simulink model "METI_CVT_Thermal_ver01_2015a"  (R2015a)
settings: Solver=ode8  SolverMode=SingleTasking  StartTime=0  StopTime=1204  FixedStep=sampling_time  RelTol=1e-3
PreLoadFcn:
  | init_setting;
values from neighbouring files (symbols this model uses):
  degC2K = 273.15    [METI_TRAMI_Thermal_ver01_Jmaab_PreLoad.m]    (also in init_setting_METI.m)
  K2degC = -273.15    [METI_TRAMI_Thermal_ver01_Jmaab_PreLoad.m]    (also in init_setting_METI.m)
  sampling_time = 0.0025    [METI_TRAMI_Thermal_ver01_Jmaab_PreLoad.m]
undefined symbols (not defined in the file or in its folder): ALT_CNT_ALT_OFF_RPM_HYS_rpm, ALT_CNT_ALT_ON_RPM_HYS_rpm, ALT_CNT_Alter_V_BASE_V, ALT_CNT_Alter_V_Kaisei_V, ALT_CNT_flag_disable_kaisei, ALT_CNT_V_Battely_Kudo_V, ALT_PNT_ALT_GDCurrent_A, ALT_PNT_ALT_GDVolt_V, ALT_PNT_Alter_limit_Current_V_table, ALT_PNT_Alter_limit_Current_V_table_x_rpm, ALT_PNT_Alter_trq_Nm_map, ALT_PNT_Alter_trq_Nm_map_x_rpm, ALT_PNT_Alter_trq_Nm_map_y_Current_A, ALT_PNT_Alter_trq_Nm_map_z_Volt_tgt_V, ALT_PNT_eta_pulley_alt, ALT_PNT_Gain_Alt_v_del, ALT_PNT_ratio_pulley_alt, ALT_PNT_Tau_Alternator_V_tgt_s, ALT_PNT_trq_alter_output_LL_Nm, BK_PNT_Pow_UL, BK_PNT_Tau_brake, Brk_LL, Brk_PGain, Brk_UL, BT_PNT_Lo_Capa_lo_batt_F, BT_PNT_Lo_ocv_SOC_lo_batt_OCV_V_table, BT_PNT_Lo_ocv_SOC_lo_batt_OCV_V_table_x_SOC, BT_PNT_Lo_R_lo_batt_ohm, BT_PNT_Lo_SOC_MAX_lo_batt, BT_PNT_Lo_SOC_MIN_lo_batt, BT_PNT_Lo_SOC_START_lo_batt, DF_PNT_DF_gear, DF_PNT_DFBlock2DFAir_Heat_Resi_KpW, DF_PNT_DFBlock_Heat_Capa_JpK, DF_PNT_DFBlock_Temp_ini_degC, DF_PNT_DFOil2DFBlock_Heat_Resi_KpW, DF_PNT_DFOil_Heat_Capa_JpK, DF_PNT_DFOil_Temp_ini_degC, DF_PNT_Driveshaft_damper, DF_PNT_Driveshaft_delta_radps_LL, DF_PNT_Driveshaft_delta_radps_UL, DF_PNT_Driveshaft_spring, DF_PNT_eta_DF, DF_PNT_Outtemp_degC, DF_PNT_TMBlock2DFBlock_Heat_Resi_KpW, Driver_Brake_Const1, Driver_Brake_Const3, Driver_Brake_Switch_Const2, Driver_Brk_sh, drivmode_ACC, drivmode_CONST, drivmode_GensokuKaisei, drivmode_GensokuRikko, drivmode_STOP, EL_PNT_R_bodyelec_lo_ohm, ENG_CNT_acc_idlestop, ENG_CNT_Accel_LL, ENG_CNT_Accel_UL, ENG_CNT_brak_idlestop, ENG_CNT_flag_idle_stop_exe ... (+133)
undefined symbols (not defined in the file): ACC_D_Gain, ACC_I_Gain, ACC_P_Gain
libraries: METI_Lib_vehicle_model x32, simulink x7, AZAPA_Lib_vehicle_model x1
(part 2 of 3)

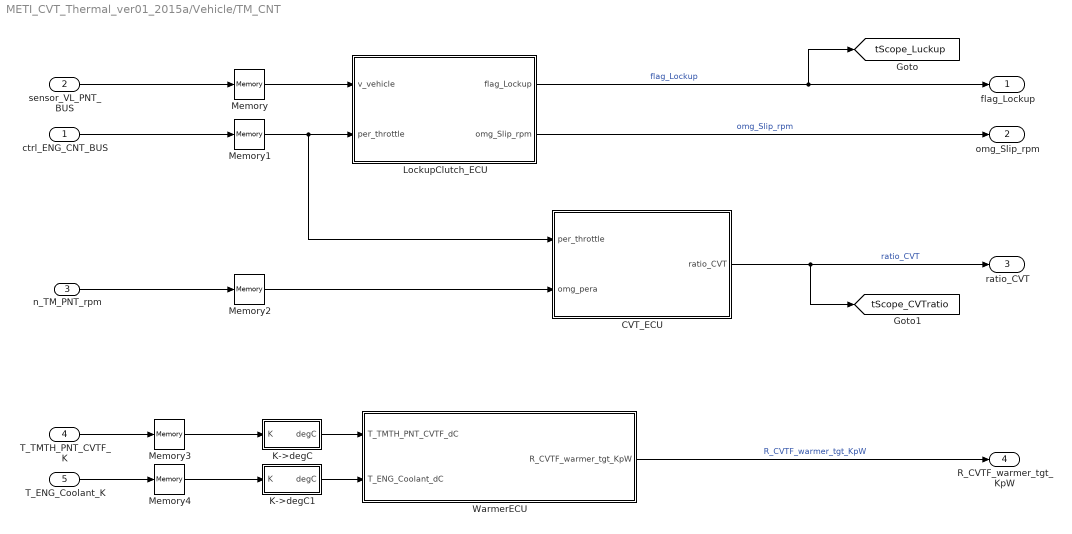
== system METI_CVT_Thermal_ver01_2015a/Vehicle/TM_CNT ==
  ctrl_ENG_CNT_BUS : Inport
  sensor_VL_PNT_BUS : Inport  Port=2
  n_TM_PNT_rpm : Inport  Port=3
  T_TMTH_PNT_CVTF_K : Inport  Port=4
  T_ENG_Coolant_K : Inport  Port=5
  CVT_ECU : Subsystem
  K->degC : Subsystem
  K->degC1 : Subsystem
  LockupClutch_ECU : Subsystem
  Memory{,1..4} (5 alike) : Memory
  WarmerECU : Subsystem
  flag_Lockup : Outport
  omg_Slip_rpm : Outport  Port=2
  ratio_CVT : Outport  Port=3
  R_CVTF_warmer_tgt_KpW : Outport  Port=4
  tag scope: tScope_CVTratio=global, tScope_Luckup=global
  wires:
  CVT_ECU/1(ratio_CVT) -> [tScope_CVTratio], ratio_CVT/1  "ratio_CVT"
  LockupClutch_ECU/1(flag_Lockup) -> [tScope_Luckup], flag_Lockup/1  "flag_Lockup"
  LockupClutch_ECU/2(omg_Slip_rpm) -> omg_Slip_rpm/1  "omg_Slip_rpm"
  ctrl_ENG_CNT_BUS/1 -> Memory1/1
  Memory/1 -> LockupClutch_ECU/1(v_vehicle)
  Memory1/1 -> CVT_ECU/1(per_throttle), LockupClutch_ECU/2(per_throttle)
  Memory2/1 -> CVT_ECU/2(omg_pera)
  n_TM_PNT_rpm/1 -> Memory2/1
  sensor_VL_PNT_BUS/1 -> Memory/1
  T_TMTH_PNT_CVTF_K/1 -> Memory3/1
  T_ENG_Coolant_K/1 -> Memory4/1
  Memory3/1 -> K->degC/1(K)
  Memory4/1 -> K->degC1/1(K)
  WarmerECU/1(R_CVTF_warmer_tgt_KpW) -> R_CVTF_warmer_tgt_KpW/1  "R_CVTF_warmer_tgt_KpW"
  K->degC/1(degC) -> WarmerECU/1(T_TMTH_PNT_CVTF_dC)
  K->degC1/1(degC) -> WarmerECU/2(T_ENG_Coolant_dC)

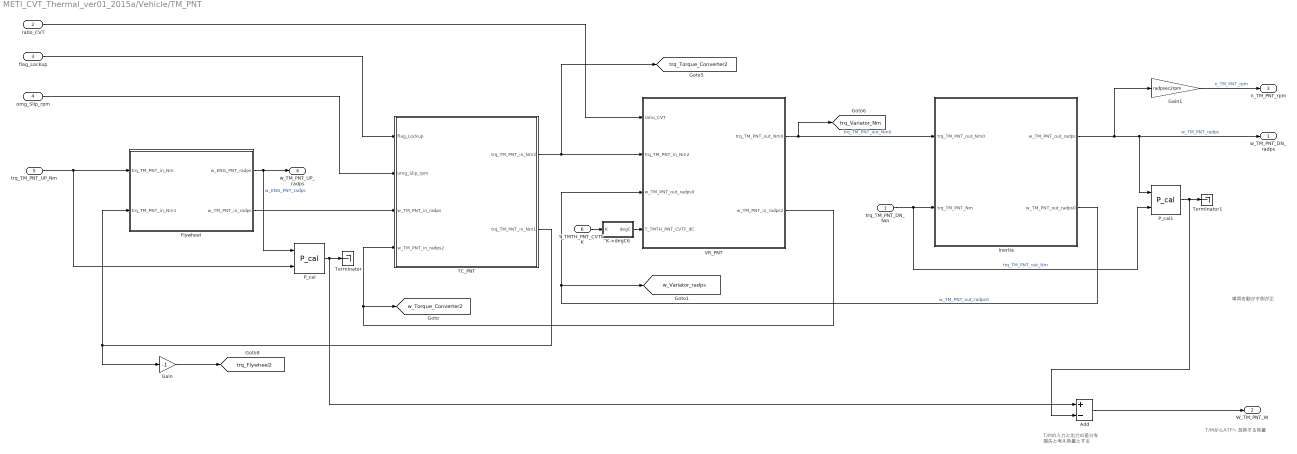
== system METI_CVT_Thermal_ver01_2015a/Vehicle/TM_PNT ==
  note: 車両を動かす側が正
  note: T/MからATFへ
      | 放熱する熱量
  note: T/Mの入力と出力の差分を
      | 損失と考え熱量とする
  trq_TM_PNT_DN_Nm : Inport
  ratio_CVT : Inport  Port=2
  flag_Lockup : Inport  Port=3
  omg_Slip_rpm : Inport  Port=4
  trq_TM_PNT_UP_Nm : Inport  Port=5
  T_TMTH_PNT_CVTF_K : Inport  Port=6
  Add : Sum  Inputs=+-
  Flywheel : Subsystem
  Gain : Gain  Gain=-1
  Gain1 : Gain  Gain=radpsec2rpm
  Inertia : Subsystem
  K->degC6 : Subsystem
  P_cal : METI_Lib_vehicle_model/P_cal  Type_energy=回転運動  Type_output_energy=出力  Power_name=Po_  t_Workspace_Name=TM_PNT_MECK_UP  P_VariableName=Po_TM_PNT_MECK_UP  Across_VariableName=w_TM_PNT_MECK_UP  Throgh_VariableName=tq_TM_PNT_MECK_UP
  P_cal1 : METI_Lib_vehicle_model/P_cal  Type_energy=回転運動  Type_output_energy=出力  Power_name=Po_  t_Workspace_Name=TM_PNT_MECK_DN  P_VariableName=Po_TM_PNT_MECK_DN  Across_VariableName=w_TM_PNT_MECK_DN  Throgh_VariableName=tq_TM_PNT_MECK_DN
  TC_PNT : Subsystem
  Terminator : Terminator
  Terminator1 : Terminator
  VR_PNT : Subsystem
  w_TM_PNT_DN_radps : Outport
  W_TM_PNT_W : Outport  Port=2
  n_TM_PNT_rpm : Outport  Port=3
  w_TM_PNT_UP_radps : Outport  Port=4
  tag scope: trq_Flywheel2=global, trq_Torque_Converter2=global, trq_Variator_Nm=global, w_Torque_Converter2=global, w_Variator_radps=global
  wires:
  VR_PNT/2(w_TM_PNT_in_radps2) -> [w_Torque_Converter2], TC_PNT/4(w_TM_PNT_in_radps2)
  TC_PNT/1(trq_TM_PNT_in_Nm2) -> [trq_Torque_Converter2], VR_PNT/2(trq_TM_PNT_in_Nm2)
  flag_Lockup/1 -> TC_PNT/1(flag_Lockup)
  omg_Slip_rpm/1 -> TC_PNT/2(omg_Slip_rpm)
  ratio_CVT/1 -> VR_PNT/1(ratio_CVT)
  TC_PNT/2(trq_TM_PNT_in_Nm1) -> Gain/1, Flywheel/2(trq_TM_PNT_in_Nm1)
  Flywheel/2(w_TM_PNT_in_radps) -> TC_PNT/3(w_TM_PNT_in_radps)
  Flywheel/1(w_ENG_PNT_radps) -> w_TM_PNT_UP_radps/1, P_cal/1  "w_ENG_PNT_radps"
  trq_TM_PNT_UP_Nm/1 -> P_cal/2, Flywheel/1(trq_TM_PNT_in_Nm)
  Inertia/1(w_TM_PNT_out_radps) -> w_TM_PNT_DN_radps/1, P_cal1/1, Gain1/1  "w_TM_PNT_radps"
  Gain1/1 -> n_TM_PNT_rpm/1  "n_TM_PNT_rpm"
  P_cal/1 -> Add/1, Terminator/1
  P_cal1/1 -> Terminator1/1, Add/2
  trq_TM_PNT_DN_Nm/1 -> P_cal1/2, Inertia/2(trq_TM_PNT_Nm)  "trq_TM_PNT_out_Nm"
  Inertia/2(w_TM_PNT_out_radps0) -> [w_Variator_radps], VR_PNT/3(w_TM_PNT_out_radps0)  "w_TM_PNT_out_radps0"
  VR_PNT/1(trq_TM_PNT_out_Nm0) -> [trq_Variator_Nm], Inertia/1(trq_TM_PNT_out_Nm0)  "trq_TM_PNT_out_Nm0"
  Add/1 -> W_TM_PNT_W/1
  T_TMTH_PNT_CVTF_K/1 -> K->degC6/1(K)
  Gain/1 -> [trq_Flywheel2]
  K->degC6/1(degC) -> VR_PNT/4(T_TMTH_PNT_CVTF_dC)

== system METI_CVT_Thermal_ver01_2015a/Vehicle/TR_PNT ==
  note: 転がり抵抗
  note: 並進⇔回転変換
  note: トルク⇔力変換
  note: omg (回転数rad/s) = v (車速m/s) / r (タイヤ半径(m))
  note: M (トルクNm) = F (力(N)） × r (タイヤ半径(m))
  note: 車両を動かす側が正
  note: 車両を動かす側が正
  trq_TR_PNT_UP_Nm : Inport
  v_VL_PNT_mps : Inport  Port=2
  Constant2 : Constant  Value=1/tire_r
  Product5 : Product  RndMeth=Zero
  Product6 : Product  RndMeth=Zero
  Q_cal1 : METI_Lib_vehicle_model/P_cal  Commented=on  Type_energy=並進運動  Type_output_energy=出力  Power_name=Po_  t_Workspace_Name=TR_PNT_MECK_DN  P_VariableName=Po_TR_PNT_MECK_DN  Across_VariableName=v_TR_PNT_MECK_DN  Throgh_VariableName=F_TR_PNT_MECK_DN
  Q_cal2 : METI_Lib_vehicle_model/P_cal  Commented=on  Type_energy=回転運動  Type_output_energy=出力  Power_name=Po_  t_Workspace_Name=TR_PNT_MECK_UP  P_VariableName=Po_TR_PNT_MECK_UP  Across_VariableName=w_TR_PNT_MECK_UP  Throgh_VariableName=tq_TR_PNT_MECK_UP
  Sum2 : Sum  Inputs=-+|
  Terminator1 : Terminator  Commented=on
  Terminator2 : Terminator  Commented=on
  cal_roll_resi : METI_Lib_vehicle_model/vehicle_model/cal_roll_resi  Myu_tire=myu  Vehicle_Mass=M  Gravi_acc=g
  w_TR_PNT_UP_radps : Outport
  F_TR_PNT_DN_N : Outport  Port=2
  wires:
  Sum2/1 -> F_TR_PNT_DN_N/1  "f_TR_PNT_N"
  cal_roll_resi/1 -> Sum2/1, Q_cal1/2
  Product6/1 -> Sum2/2
  Q_cal1/1 -> Terminator1/1
  Constant2/1 -> Product6/1, Product5/2
  v_VL_PNT_mps/1 -> cal_roll_resi/1, Q_cal1/1, Product5/1
  Q_cal2/1 -> Terminator2/1
  Product5/1 -> Q_cal2/1, w_TR_PNT_UP_radps/1  "w_TR_PNT_radps"
  trq_TR_PNT_UP_Nm/1 -> Q_cal2/2, Product6/2

== system METI_CVT_Thermal_ver01_2015a/Vehicle/VL_PNT ==
  note: 空気抵抗
  note: 車両慣性
  note: 登坂抵抗
  note: 車両を動かす側が正
  F_VL_PNT_N : Inport
  Constant1 : Constant  Value=VL_PNT_Vehicle_Const
  Product2 : Product
  Q_cal2 : METI_Lib_vehicle_model/P_cal  Type_energy=並進運動  Type_output_energy=出力  Power_name=Po_  t_Workspace_Name=VL_PNT_MASS_MECK  P_VariableName=Po_VL_PNT_MASS_MECK  Across_VariableName=v_VL_PNT_MASS_MECK  Throgh_VariableName=F_VL_PNT_MASS_MECK
  Q_cal3 : METI_Lib_vehicle_model/P_cal  Type_energy=並進運動  Type_output_energy=出力  Power_name=Po_  t_Workspace_Name=VL_PNT_MECK  P_VariableName=Po_VL_PNT_MECK  Across_VariableName=v_VL_PNT_MECK  Throgh_VariableName=F_VL_PNT_MECK
  Q_cal4 : METI_Lib_vehicle_model/P_cal  Type_energy=並進運動  Type_output_energy=損失  Power_name=Pl_  t_Workspace_Name=VL_PNT_Airresi_MECK_LOSS  P_VariableName=Pl_VL_PNT_Airresi_MECK_LOSS  Across_VariableName=v_VL_PNT_Airresi_MECK_LOSS  Throgh_VariableName=F_VL_PNT_Airresi_MECK_LOSS
  Sum1 : Sum  Inputs=-+|
  Sum3 : Sum  Inputs=-+|
  Terminator2 : Terminator
  Terminator3 : Terminator
  Terminator4 : Terminator  Commented=on
  To Workspace3 : ToWorkspace  VariableName=Q_GradrResi  SaveFormat=Structure With Time  SampleTime=-1
      settings: Decimation=100
  V_wind : Constant  Value=VL_PNT_V_wind
  cal_Air_resi : METI_Lib_vehicle_model/vehicle_model/cal_Air_resi  Vel_max=vel_max
  cal_Vehicle_Mass : METI_Lib_vehicle_model/vehicle_model/cal_Vehicle_Mass  Vehicle_Mass=M
  mps2kmph : Gain  Gain=mps2kmph
  v_VL_PNT_kmph : Outport
  v_VL_PNT_mps : Outport  Port=2
  tag scope: v_VL_PNT_mps=global
  wires:
  Product2/1 -> To Workspace3/1
  Sum3/1 -> Sum1/2
  Sum1/1 -> Q_cal2/2, cal_Vehicle_Mass/1
  cal_Vehicle_Mass/1 -> mps2kmph/1, Q_cal3/1, cal_Air_resi/1, Q_cal4/1, Product2/1, v_VL_PNT_mps/1, [v_VL_PNT_mps], Q_cal2/1  "v_VL_PNT_mps"
  cal_Air_resi/1 -> Q_cal4/2, Sum3/1
  V_wind/1 -> cal_Air_resi/2
  Constant1/1 -> Product2/2, Sum1/1
  Q_cal2/1 -> Terminator2/1
  Q_cal3/1 -> Terminator3/1
  Q_cal4/1 -> Terminator4/1
  mps2kmph/1 -> v_VL_PNT_kmph/1  "v_VL_PNT_kmph"
  F_VL_PNT_N/1 -> Sum3/2, Q_cal3/2

== system METI_CVT_Thermal_ver01_2015a/Driver/Caliculate_Opeining_Accel/FB ==
  delta_v_VL_kmph : Inport
  Acc_D_Gain : Gain  Gain=D_Gain
  Acc_I_Gain : Gain  Gain=I_Gain
  Acc_P_Gain : Gain  Gain=P_Gain
  Acc_P_Gain1 : Gain  Gain=P_Gain
  Derivative : Derivative
  Filter : Subsystem  Commented=through
  Integrator : Integrator
  Memory : Memory
  Product1 : Product
  Saturation2 : Saturate  UpperLimit=1  LowerLimit=0
  Sum : Sum  Inputs=+++
  Terminator : Terminator
  FB_open_accel_per : Outport
  wires:
  Filter/1(Out1) -> Product1/2
  Saturation2/1 -> Acc_P_Gain/1
  Acc_P_Gain/1 -> Product1/1
  Sum/1 -> FB_open_accel_per/1
  Derivative/1 -> Acc_D_Gain/1
  Integrator/1 -> Acc_I_Gain/1
  delta_v_VL_kmph/1 -> Memory/1
  Acc_I_Gain/1 -> Sum/3
  Acc_D_Gain/1 -> Sum/2
  Product1/1 -> Sum/1
  Memory/1 -> Saturation2/1, Filter/1(In1), Acc_P_Gain1/1, Integrator/1, Derivative/1
  Acc_P_Gain1/1 -> Terminator/1

== system METI_CVT_Thermal_ver01_2015a/Driver/Caliculate_Opeining_Accel/FF ==
  note: 速度とパワーでF/B出来るようにモデルを用意しておく
      | 切り替えスイッチを作っておく
  v_VL_PNT_kmph : Inport
  target_v_VL_kmph : Inport  Port=2
  pre_n_eng_rpm : Inport  Port=3
  pre_ratio_CVT : Inport  Port=4
  Air_Resistance : Subsystem
  Cal_M_ENG_jiku2 : Subsystem
  Constant1 : Constant  Value=TM_CNT_CVT_ratio_LL
  Constant3 : Constant  Value=tire_r
  Constant4 : Constant  Value=DF_PNT_DF_gear
  Inertial_Resistance : Subsystem
  MinMax : MinMax  Function=max  Inputs=2
  Product8 : Product  Inputs=*/*/  RndMeth=Zero
  Rolling_Resistance : Subsystem
  Sum4 : Sum  Inputs=+++
  Terminator : Terminator
  Transfer Fcn : TransferFcn  Denominator=[TM_PNT_Tau_CVT_ratio_s 1]
  kmph2mps : Gain  Gain=kmph2mps
  kmph2mps1 : Gain  Gain=kmph2mps
  FF_open_accel_per : Outport
  wires:
  kmph2mps/1 -> Inertial_Resistance/1(V_tgt), Rolling_Resistance/1(V_tgt), Air_Resistance/1(V_tgt)
  target_v_VL_kmph/1 -> kmph2mps/1
  Sum4/1 -> Product8/1
  Constant4/1 -> Product8/2
  Constant3/1 -> Product8/3
  Air_Resistance/1(F_air_resi) -> Sum4/2
  Rolling_Resistance/1(F_rollresi) -> Sum4/3
  Inertial_Resistance/1(F_Inertia) -> Sum4/1
  pre_ratio_CVT/1 -> Transfer Fcn/1
  Constant1/1 -> MinMax/2
  MinMax/1 -> Product8/4
  Transfer Fcn/1 -> MinMax/1
  v_VL_PNT_kmph/1 -> kmph2mps1/1
  kmph2mps1/1 -> Terminator/1
  Cal_M_ENG_jiku2/1(FF_open_accel_per) -> FF_open_accel_per/1
  Product8/1 -> Cal_M_ENG_jiku2/1(FF_trq_accel_Nm)  "FF_trq_accel_Nm"
  pre_n_eng_rpm/1 -> Cal_M_ENG_jiku2/2(pre_n_eng_rpm)

== system METI_CVT_Thermal_ver01_2015a/Vehicle/ALT_PNT/Subsystem ==
  note: V_ALT_PNT
  note: オルタ要求トルク上限/下限ガード処理追加
      | (低回転数、低電流時に要求トルクが過大となるのを防止するため
      |  :マップの外挿方法が線形となっていることが原因)
  target_volt_ALT_V : Inport
  w_ROT_slavepulley12 : Inport  Port=2
  volt_BT_PNT_Lo_V : Inport  Port=3
  Constant1 : Constant  Value=ALT_PNT_ALT_GDCurrent_A
  Constant2 : Constant  Value=ALT_PNT_ALT_GDVolt_V
  I_alt_cal : Subsystem
  Torque_Guard : Subsystem
  Transfer Fcn1 : TransferFcn  Denominator=|
      | [ALT_PNT_Tau_Alternator_trq_Nm
      |  1]
  omg2rpm : Gain  Gain=radpsec2rpm
  current_ALT_PNT_A : Outport
  trq_trqsource : Outport  Port=2
  wires:
  I_alt_cal/1(I_alt) -> Torque_Guard/1(current_ALT_PNT_A), current_ALT_PNT_A/1  "current_ALT_PNT_A"
  target_volt_ALT_V/1 -> I_alt_cal/1(target_volt_ALT_V)
  volt_BT_PNT_Lo_V/1 -> Torque_Guard/2(V_ALT_PNT), I_alt_cal/2(volt_BT_PNT_Lo_V)
  Transfer Fcn1/1 -> trq_trqsource/1
  omg2rpm/1 -> Torque_Guard/3(n_ROT_slavepulley12_rpm), I_alt_cal/3(rpm_alt)  "n_ROT_slavepulley12_rpm"
  w_ROT_slavepulley12/1 -> omg2rpm/1
  Constant1/1 -> Torque_Guard/4(ALT_GDCurrent)
  Constant2/1 -> Torque_Guard/5(ALT_GDVolt)
  Torque_Guard/1(trq_trqsource) -> Transfer Fcn1/1

== system METI_CVT_Thermal_ver01_2015a/Vehicle/ALT_PNT/pulley_slave ==
  note: プーリー比
  note: プーリー効率
  w_ENG_PNT_radps : Inport
  trq_slavepulley12 : Inport  Port=2
  P_cal : AZAPA_Lib_vehicle_model/P_cal  Commented=on  Type_energy=並進運動  Type_output_energy=出力  Power_name=Po_  t_Workspace_Name=MOTOR_MECK  P_VariableName=Po_MOTOR_MECK  Across_VariableName=v_MOTOR_MECK  Throgh_VariableName=F_MOTOR_MECK
  P_cal1 : METI_Lib_vehicle_model/P_cal  Type_energy=回転運動  Type_output_energy=損失  Power_name=Pl_  t_Workspace_Name=ALT_PNT_Pulley  P_VariableName=Pl_ALT_PNT_Pulley  Across_VariableName=w_ALT_PNT_Pulley  Throgh_VariableName=tq_ALT_PNT_Pulley
  Product : Product  RndMeth=Zero
  Product1 : Product  RndMeth=Zero
  eta_cal2 : METI_Lib_vehicle_model/eta_cal2
  eta_pulley : Constant  Value=ALT_PNT_eta_pulley_alt
  ratio_pulley : Constant  Value=ALT_PNT_ratio_pulley_alt
  trq_slavepulley11 : Outport
  w_slavepulley12 : Outport  Port=2
  tag scope: tScope_pulley1Loss=global
  wires:
  eta_cal2/1 -> P_cal1/2
  P_cal1/1 -> [tScope_pulley1Loss]
  w_ENG_PNT_radps/1 -> P_cal1/1, Product1/1
  eta_cal2/2 -> trq_slavepulley11/1
  trq_slavepulley12/1 -> Product/2
  eta_pulley/1 -> eta_cal2/1
  Product1/1 -> w_slavepulley12/1
  ratio_pulley/1 -> Product/1, Product1/2
  Product/1 -> eta_cal2/2

== system METI_CVT_Thermal_ver01_2015a/Vehicle/ATM_PNT/degC->K ==
  degC : Inport
  Constant2 : Constant  Value=degC2K
  Sum : Sum  Inputs=++|
  K : Outport
  wires:
  degC/1 -> Sum/2
  Constant2/1 -> Sum/1
  Sum/1 -> K/1

== system METI_CVT_Thermal_ver01_2015a/Vehicle/ATM_PNT/degC->K1 ==
  degC : Inport
  Constant2 : Constant  Value=degC2K
  Sum : Sum  Inputs=++|
  K : Outport
  wires:
  Sum/1 -> K/1
  Constant2/1 -> Sum/1
  degC/1 -> Sum/2

== system METI_CVT_Thermal_ver01_2015a/Vehicle/ATM_PNT/degC->K2 ==
  degC : Inport
  Constant2 : Constant  Value=degC2K
  Sum : Sum  Inputs=++|
  K : Outport
  wires:
  degC/1 -> Sum/2
  Constant2/1 -> Sum/1
  Sum/1 -> K/1

== system METI_CVT_Thermal_ver01_2015a/Vehicle/ATM_PNT/degC->K3 ==
  degC : Inport
  Constant2 : Constant  Value=degC2K
  Sum : Sum  Inputs=++|
  K : Outport
  wires:
  Sum/1 -> K/1
  Constant2/1 -> Sum/1
  degC/1 -> Sum/2

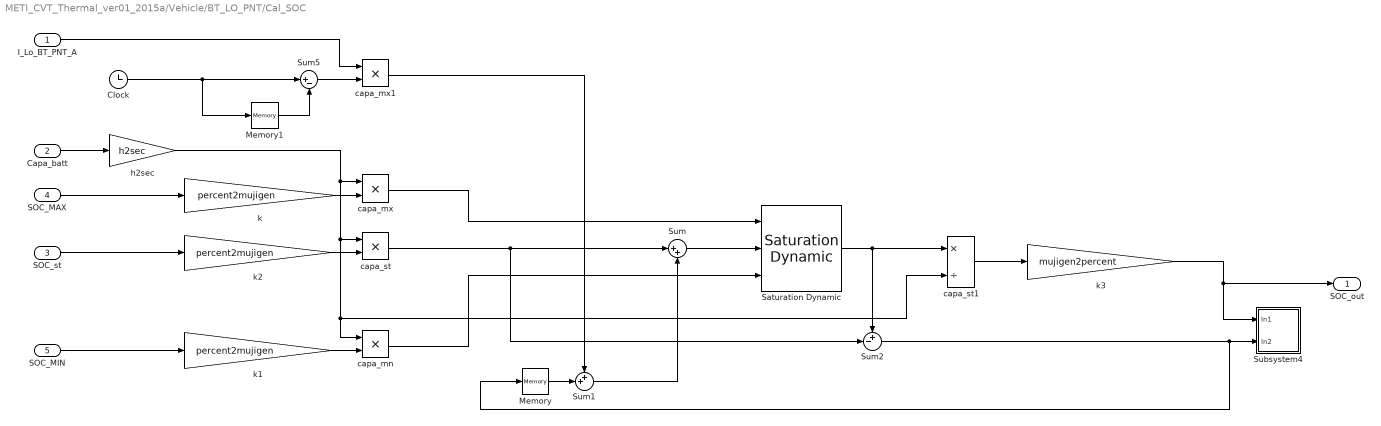
== system METI_CVT_Thermal_ver01_2015a/Vehicle/BT_LO_PNT/Cal_SOC ==
  I_Lo_BT_PNT_A : Inport
  Capa_batt : Inport  Port=2
  SOC_st : Inport  Port=3
  SOC_MAX : Inport  Port=4
  SOC_MIN : Inport  Port=5
  Clock : Clock
  Memory : Memory
  Memory1 : Memory
  Saturation Dynamic : simulink/Discontinuities/Saturation Dynamic  OutMin=[]  OutMax=[]  OutDataTypeStr=Inherit: Same as second input  OutDataType=fixdt(1, 16)  OutScaling=2^-10  DoSatur=off
  Subsystem4 : Subsystem  mask{SOC=SOC_LoBat, VariableName=Asec_LoBat}
      mask prompts: SOC "バッテリSOC"; VariableName "バッテリ容量変化量(Asec)"
  Sum : Sum  Inputs=|++
  Sum1 : Sum  Inputs=++|
  Sum2 : Sum  Inputs=+-|
  Sum5 : Sum  Inputs=|+-
  capa_mn : Product  RndMeth=Zero
  capa_mx : Product  RndMeth=Zero
  capa_mx1 : Product  RndMeth=Zero
  capa_st : Product  RndMeth=Zero
  capa_st1 : Product  Inputs=*/  RndMeth=Zero
  h2sec : Gain  Gain=h2sec
  k : Gain  Gain=percent2mujigen
  k1 : Gain  Gain=percent2mujigen
  k2 : Gain  Gain=percent2mujigen
  k3 : Gain  Gain=mujigen2percent
  SOC_out : Outport
  wires:
  Sum5/1 -> capa_mx1/2
  Memory1/1 -> Sum5/2
  Sum/1 -> Saturation Dynamic/2
  Clock/1 -> Sum5/1, Memory1/1
  capa_mx1/1 -> Sum1/1
  k3/1 -> Subsystem4/1(In1), SOC_out/1
  Sum1/1 -> Sum/2
  Memory/1 -> Sum1/2
  k2/1 -> capa_st/2
  k1/1 -> capa_mn/2
  k/1 -> capa_mx/2
  capa_st/1 -> Sum2/2, Sum/1
  Saturation Dynamic/1 -> Sum2/1, capa_st1/1
  capa_mx/1 -> Saturation Dynamic/1
  capa_mn/1 -> Saturation Dynamic/3
  capa_st1/1 -> k3/1
  h2sec/1 -> capa_mn/1, capa_st1/2, capa_st/1, capa_mx/1
  SOC_MIN/1 -> k1/1
  SOC_MAX/1 -> k/1
  SOC_st/1 -> k2/1
  Capa_batt/1 -> h2sec/1
  I_Lo_BT_PNT_A/1 -> capa_mx1/1
  Sum2/1 -> Memory/1, Subsystem4/2(In2)

== system METI_CVT_Thermal_ver01_2015a/Vehicle/BT_LO_PNT/Subsystem ==
  I_BT_PNT_Lo_A : Inport
  Divide : Product
  Resistivity : Constant  Value=BT_PNT_Lo_R_lo_batt_ohm
  Sum : Sum  Inputs=|++
  Transfer Fcn : TransferFcn  Numerator=[0.01]  Denominator=[0.1 1]
  V_BT_PNT_Lo_V : Outport
  wires:
  Resistivity/1 -> Divide/2
  Divide/1 -> Sum/1
  I_BT_PNT_Lo_A/1 -> Divide/1, Transfer Fcn/1
  Sum/1 -> V_BT_PNT_Lo_V/1
  Transfer Fcn/1 -> Sum/2

== system METI_CVT_Thermal_ver01_2015a/Vehicle/DF_PNT/DriveShaft ==
  note: ドライブシャフトモデル
      | 硬いバネダンパー
  w_TR_PNT_radps : Inport
  w_DS_PNT_in_radps : Inport  Port=2
  Gain : Gain  Gain=-1
  Gain1 : Gain  Gain=DF_PNT_Driveshaft_spring
  Gain2 : Gain  Gain=DF_PNT_Driveshaft_damper
  Integrator : Integrator  LimitOutput=on  UpperSaturationLimit=DF_PNT_Driveshaft_delta_radps_UL  LowerSaturationLimit=DF_PNT_Driveshaft_delta_radps_LL
  Sum : Sum  Inputs=|+-
  Sum2 : Sum  Inputs=|++
  trq_DS_PNT_in_Nm : Outport
  trq_DF_PNT_Nm : Outport  Port=2
  wires:
  w_TR_PNT_radps/1 -> Sum/2
  w_DS_PNT_in_radps/1 -> Sum/1
  Integrator/1 -> Gain1/1
  Sum/1 -> Integrator/1, Gain2/1
  Gain1/1 -> Sum2/1
  Gain2/1 -> Sum2/2
  Sum2/1 -> Gain/1, trq_DS_PNT_in_Nm/1
  Gain/1 -> trq_DF_PNT_Nm/1

== system METI_CVT_Thermal_ver01_2015a/Vehicle/ENG_CNT/Caliculate_Idle_Speed ==
  note: 目標アイドル回転数
  note: ○目標回転数に対するP制御
  note: 補機負荷やNDの時の負荷によるアイドル安定化処理を入れる
      | パワーデマンドで締結
  per_throttle_base : Inport
  n_eng_rpm : Inport  Port=2
  flag_Lockup : Inport  Port=3
  flag_IdleStop : Inport  Port=4
  T_ENGTH_PNT_Coolant_dC : Inport  Port=5
  Subsystem : Subsystem
  Subsystem1 : Subsystem
  Subtract : Sum  Inputs=+-
  Tw2ENG_CNT_IdleSpeed : Lookup_n-D  NumberOfTableDimensions=1  BreakpointsForDimension1=T_ENGCoodant_T_ENGCoodant  Table=ENG_CNT_IdleSpeed  InternalRulePriority=Speed  RndMeth=Simplest  InputSameDT=on
  per_isc_[%] : Outport
  tag scope: ENG_CNT_IdleSpeed=global
  wires:
  n_eng_rpm/1 -> Subsystem1/2(n_eng_rpm), Subtract/2
  Subtract/1 -> Subsystem/1(del_omg_engine)
  per_throttle_base/1 -> Subsystem1/3(per_throttle_base)
  flag_Lockup/1 -> Subsystem1/4(flag_Lockup)
  Subsystem1/1(flag_idle_fb) -> Subsystem/2(flag_idle_fb)
  flag_IdleStop/1 -> Subsystem1/5(flag_IdleStop)
  Subsystem/1(per_isc_[%]) -> per_isc_[%]/1
  T_ENGTH_PNT_Coolant_dC/1 -> Tw2ENG_CNT_IdleSpeed/1
  Tw2ENG_CNT_IdleSpeed/1 -> [ENG_CNT_IdleSpeed], Subsystem1/1(omg_tgt_idle), Subtract/1

== system METI_CVT_Thermal_ver01_2015a/Vehicle/ENG_CNT/Injection_Control ==
  T_ENGTH_PNT_Coolant_dC : Inport
  Tw2KFuel : Lookup_n-D  NumberOfTableDimensions=1  BreakpointsForDimension1=T_ENGCoodant  Table=K_Fuel  RndMeth=Simplest  InputSameDT=on
  K_Fuel : Outport
  wires:
  Tw2KFuel/1 -> K_Fuel/1  "K_Fuel"
  T_ENGTH_PNT_Coolant_dC/1 -> Tw2KFuel/1

== system METI_CVT_Thermal_ver01_2015a/Vehicle/ENG_CNT/K->degC7 ==
  K : Inport
  Constant2 : Constant  Value=K2degC
  Sum : Sum  Inputs=++|
  degC : Outport
  wires:
  Sum/1 -> degC/1
  Constant2/1 -> Sum/1
  K/1 -> Sum/2

== system METI_CVT_Thermal_ver01_2015a/Vehicle/ENG_CNT/RD_Fan_Control ==
  T_ENGTH_PNT_Coolant_dC : Inport
  1-D Lookup Table1 : Lookup_n-D  NumberOfTableDimensions=1  BreakpointsForDimension1=ENG_CNT_V_RDFan_x_T_Coolant  BeginIndexSearchUsingPreviousIndexResult=on  Table=ENG_CNT_V_RDFan_V  InternalRulePriority=Speed  RndMeth=Simplest  InputSameDT=on
  V_RDTH_PNT_Fan_V : Outport
  wires:
  T_ENGTH_PNT_Coolant_dC/1 -> 1-D Lookup Table1/1
  1-D Lookup Table1/1 -> V_RDTH_PNT_Fan_V/1

== system METI_CVT_Thermal_ver01_2015a/Vehicle/ENG_CNT/Set_Fuel_Cut ==
  note: ○減速時のフューエルカット条件
      | 　・停車中でない
      | 　・回転数がある回転数以上
      | 　・アクセル開度がOFF
  v_vehicle : Inport
  n_eng_rpm : Inport  Port=2
  per_throttle_base : Inport  Port=3
  Constant1 : Constant  Value=ENG_CNT_V_vhicle_fuelcut_kmph
  Constant4 : Constant  Value=ENG_CNT_omg_eng_fuelcut_rpm
  Constant6 : Constant  Value=ENG_CNT_per_throttle_fuelcut
  Logical Operator : Logic  Inputs=3  AllPortsSameDT=off  OutDataTypeStr=boolean
  Relational Operator1 : RelationalOperator  Operator=<=  OutDataTypeStr=boolean
  Relational Operator2 : RelationalOperator  OutDataTypeStr=boolean
  Relational Operator3 : RelationalOperator  OutDataTypeStr=boolean
  flag_fuelcut : Outport
  wires:
  n_eng_rpm/1 -> Relational Operator2/1
  per_throttle_base/1 -> Relational Operator1/1
  Constant6/1 -> Relational Operator1/2
  Relational Operator1/1 -> Logical Operator/3
  Relational Operator2/1 -> Logical Operator/2
  Logical Operator/1 -> flag_fuelcut/1
  Constant1/1 -> Relational Operator3/2
  v_vehicle/1 -> Relational Operator3/1
  Relational Operator3/1 -> Logical Operator/1
  Constant4/1 -> Relational Operator2/2

== system METI_CVT_Thermal_ver01_2015a/Vehicle/ENG_CNT/Set_Idle_Stop ==
  note: ○アイドリングストップ制御
      | 　停車時＋ブレーキを踏んでいるとき、アイドリングストップ
  open_accel_per : Inport
  v_vehicle : Inport  Port=2
  per_brake : Inport  Port=3
  T_ENGTH_PNT_Coolant_dC : Inport  Port=4
  Constant : Constant  Value=ENG_CNT_V_car_idlestop_kmph
  Constant1 : Constant  Value=ENG_CNT_brak_idlestop
  Constant2 : Constant  Value=ENG_CNT_flag_idle_stop_exe
  Constant3 : Constant  Value=ENG_CNT_acc_idlestop
  Logical Operator : Logic  Inputs=5  AllPortsSameDT=off  OutDataTypeStr=boolean
  Relational Operator : RelationalOperator  Operator=<  OutDataTypeStr=boolean
  Relational Operator1 : RelationalOperator  OutDataTypeStr=boolean
  Relational Operator2 : RelationalOperator  Operator=<  OutDataTypeStr=boolean
  Relay : Relay  OnSwitchValue=ENG_CNT_IdleStop_flag_const  OffSwitchValue=ENG_CNT_IdleStop_flag_const-5
  flag_IdleStop : Outport
  wires:
  Relational Operator/1 -> Logical Operator/2
  Logical Operator/1 -> flag_IdleStop/1
  v_vehicle/1 -> Relational Operator/1
  per_brake/1 -> Relational Operator1/1
  Constant/1 -> Relational Operator/2
  Constant1/1 -> Relational Operator1/2
  Relational Operator1/1 -> Logical Operator/3
  Constant2/1 -> Logical Operator/1
  T_ENGTH_PNT_Coolant_dC/1 -> Relay/1
  Relay/1 -> Logical Operator/4
  open_accel_per/1 -> Relational Operator2/1
  Constant3/1 -> Relational Operator2/2
  Relational Operator2/1 -> Logical Operator/5

== system METI_CVT_Thermal_ver01_2015a/Vehicle/ENG_CNT/Starter ==
  note: サンプリング時間
  note: 時間リセット
  note: アイドリングフラグがON→OFFに
      | 切り替わり時スターターON開始
  note: スタータ開始時間
  note: スタータ開始時間から
      | ある時間超えたらOFF
  note: アイドリングフラグがON→OFFに切り替わり時スターターON開始.ある時間を超えたらOFF
  flag_idlestop : Inport
  n_eng_rpm : Inport  Port=2
  Constant2 : Constant  Value=ENG_CNT_Starter_timer_Const_s
  Constant4 : Constant  Value=sampling_time
  Constant5 : Constant  Value=0
  Constant6 : Constant  Value=OFF
  Constant7 : Constant  Value=ON
  IdleSpeed : Constant  Value=ENG_CNT_IdleSpeed_Const/2
  Logical Operator : Logic  Inputs=3  AllPortsSameDT=off  OutDataTypeStr=boolean
  Logical Operator1 : Logic  Operator=NOT  AllPortsSameDT=off  OutDataTypeStr=boolean
  Memory : Memory  X0=1000
  Memory1 : Memory  InheritSampleTime=on
  Relational Operator1 : RelationalOperator  Operator=<=  OutDataTypeStr=boolean
  Relational Operator2 : RelationalOperator  Operator=<  OutDataTypeStr=boolean
  Sum5 : Sum  Inputs=|++
  Switch3 : Switch  Criteria=u2 > Threshold  Threshold=0.5
  Switch4 : Switch  Criteria=u2 > Threshold  Threshold=0.5
  flag_ON_Starter : Outport
  wires:
  Switch4/1 -> flag_ON_Starter/1
  Memory/1 -> Sum5/2
  Constant4/1 -> Sum5/1
  Constant5/1 -> Switch3/1
  Sum5/1 -> Switch3/3
  Switch3/1 -> Relational Operator1/1, Memory/1
  Memory1/1 -> Logical Operator/2
  Logical Operator1/1 -> Logical Operator/1
  flag_idlestop/1 -> Memory1/1, Logical Operator1/1
  Logical Operator/1 -> Switch3/2
  Constant2/1 -> Relational Operator1/2
  Relational Operator1/1 -> Switch4/2
  Constant7/1 -> Switch4/1
  Constant6/1 -> Switch4/3
  n_eng_rpm/1 -> Relational Operator2/1
  IdleSpeed/1 -> Relational Operator2/2
  Relational Operator2/1 -> Logical Operator/3

== system METI_CVT_Thermal_ver01_2015a/Vehicle/ENG_CNT/Water_Pump_Control ==
  T_ENGTH_PNT_Coolant_dC : Inport
  1-D Lookup Table1 : Lookup_n-D  NumberOfTableDimensions=1  BreakpointsForDimension1=ENG_CNT_V_Water_Pump_x_T_Coolant  BeginIndexSearchUsingPreviousIndexResult=on  Table=ENG_CNT_V_Water_Pump_V  InternalRulePriority=Speed  RndMeth=Simplest  InputSameDT=on
  V_ENG_PNT_WP_V : Outport
  wires:
  T_ENGTH_PNT_Coolant_dC/1 -> 1-D Lookup Table1/1
  1-D Lookup Table1/1 -> V_ENG_PNT_WP_V/1

== system METI_CVT_Thermal_ver01_2015a/Vehicle/ENG_PNT/Cal_FuelComsunption ==
  w_ENG_PNT_radps : Inport
  trq_ENG : Inport  Port=2
  flag_fuelcut : Inport  Port=3
  flag_IdleStop : Inport  Port=4
  timing_ignition : Inport  Port=5
  K_Fuel : Inport  Port=6
  1-D Lookup Table1 : Lookup_n-D  NumberOfTableDimensions=1  BreakpointsForDimension1=ENG_PNT_trq_fluc_Nm_table_x_spk_tim  Table=ENG_PNT_trq_fluc_Nm_table  RndMeth=Simplest  InputSameDT=on
  Map_FuelRate : Lookup_n-D  BreakpointsForDimension1=ENG_PNT_FuelCon_gps_map_y_trq_Nm  BreakpointsForDimension2=ENG_PNT_FuelCon_gps_map_x_pri_rpm  Table=ENG_PNT_FuelCon_gps_map  RndMeth=Simplest  InputSameDT=on
  Not_cal1 : Subsystem
  Not_cal2 : Subsystem
  Product : Product  Inputs=4  RndMeth=Zero
  Product1 : Product  Inputs=*/  RndMeth=Zero
  radpsec2rpm : Gain  Gain=radpsec2rpm
  FuelConsumption : Outport
  wires:
  trq_ENG/1 -> Product1/1
  radpsec2rpm/1 -> Map_FuelRate/2
  w_ENG_PNT_radps/1 -> radpsec2rpm/1
  Product/1 -> FuelConsumption/1
  Not_cal2/1(Out1) -> Product/3
  Not_cal1/1(Out1) -> Product/2
  flag_fuelcut/1 -> Not_cal1/1(In1)
  flag_IdleStop/1 -> Not_cal2/1(In1)
  timing_ignition/1 -> 1-D Lookup Table1/1
  1-D Lookup Table1/1 -> Product1/2
  Product1/1 -> Map_FuelRate/1
  Map_FuelRate/1 -> Product/1
  K_Fuel/1 -> Product/4

== system METI_CVT_Thermal_ver01_2015a/Vehicle/ENG_PNT/Cal_trq_ENG_jiku ==
  note: エンジン軸トルクマップ
  open_throttle_per : Inport
  flag_fuelcut : Inport  Port=2
  flag_IdleStop : Inport  Port=3
  timing_ignition : Inport  Port=4
  w_ENG_PNT_radps : Inport  Port=5
  1-D Lookup Table : Lookup_n-D  NumberOfTableDimensions=1  BreakpointsForDimension1=ENG_PNT_trq_fluc_Nm_table_x_spk_tim  Table=ENG_PNT_trq_fluc_Nm_table  RndMeth=Simplest  InputSameDT=on
  2-D Lookup Table : Lookup_n-D  BreakpointsForDimension1=ENG_PNT_trq_Nm_map_y_throttle  BreakpointsForDimension2=ENG_PNT_trq_Nm_map_x_rpm  Table=ENG_PNT_trq_Nm_map  ExtrapMethod=Clip  UseLastTableValue=on  RndMeth=Simplest  InputSameDT=on
  Model Info : simulink/Model-Wide Utilities/Model Info  Frame=on  DisplayStringWithTags=|  HorizontalTextAlignment=Left  LeftAlignmentValue=0.02  SourceBlockDiagram=METI_CVT_Thermal_ver01_2015a  TagMaxNumber=20
      | 【注記】
      | ・燃料カット時はスロットル開度を0としてエンジンフリクションを付加
      | ・点火タイミングによるトルク変動を想定
      | ・エンジン軸トルクマップの使用
  Not_cal : Subsystem
  Not_cal1 : Subsystem
  Product : Product  RndMeth=Zero
  Product1 : Product  RndMeth=Zero
  Product2 : Product  RndMeth=Zero
  Saturation : Saturate  UpperLimit=ENG_CNT_Throttle_UL  LowerLimit=ENG_CNT_Throttle_LL
  radpsec2rpm : Gain  Gain=radpsec2rpm
  trq_ENG_PNT_Nm : Outport
  wires:
  w_ENG_PNT_radps/1 -> radpsec2rpm/1
  2-D Lookup Table/1 -> Product1/1
  open_throttle_per/1 -> Product/1
  Saturation/1 -> 2-D Lookup Table/1
  radpsec2rpm/1 -> 2-D Lookup Table/2
  timing_ignition/1 -> 1-D Lookup Table/1
  1-D Lookup Table/1 -> Product1/2
  Product/1 -> Saturation/1
  Product2/1 -> Product/2
  flag_fuelcut/1 -> Not_cal/1(In1)
  Not_cal/1(Out1) -> Product2/1
  flag_IdleStop/1 -> Not_cal1/1(In1)
  Not_cal1/1(Out1) -> Product2/2
  Product1/1 -> trq_ENG_PNT_Nm/1  "trq_ENG_PNT_Nm"

== system METI_CVT_Thermal_ver01_2015a/Vehicle/ENG_PNT/Coldstart_Additional_friction_calc2 ==
  note: スロットル開度0の時の
      | 軸トルクを読み出し
  T_ENGOil_degC : Inport
  w_ENG_PNT_radps : Inport  Port=2
  1-D Lookup Table : Lookup_n-D  NumberOfTableDimensions=1  BreakpointsForDimension1=ENG_PNT_Cold_friction_gain_x_T_ENGOil  Table=ENG_PNT_Cold_friction_gain  InternalRulePriority=Speed  RndMeth=Simplest  InputSameDT=on
  2-D Lookup Table : Lookup_n-D  BreakpointsForDimension1=ENG_PNT_trq_Nm_map_y_throttle  BreakpointsForDimension2=ENG_PNT_trq_Nm_map_x_rpm  Table=ENG_PNT_trq_Nm_map  ExtrapMethod=Clip  UseLastTableValue=on  RndMeth=Simplest  InputSameDT=on
  Add : Sum  Inputs=+-
  Constant1 : Constant  Value=0
  Product : Product
  radpsec2rpm : Gain  Gain=radpsec2rpm
  Additional_friction : Outport
  wires:
  T_ENGOil_degC/1 -> 1-D Lookup Table/1
  w_ENG_PNT_radps/1 -> radpsec2rpm/1
  radpsec2rpm/1 -> 2-D Lookup Table/2
  Constant1/1 -> 2-D Lookup Table/1
  2-D Lookup Table/1 -> Add/2, Product/2
  1-D Lookup Table/1 -> Product/1
  Add/1 -> Additional_friction/1
  Product/1 -> Add/1

== system METI_CVT_Thermal_ver01_2015a/Vehicle/ENG_PNT/Coldstart_Heat_flux_gain_calc ==
  T_ENGOil_degC : Inport
  1-D Lookup Table : Lookup_n-D  NumberOfTableDimensions=1  BreakpointsForDimension1=ENG_PNT_Heatflux2ENGOil_gain_x_T_ENGOil  Table=ENG_PNT_Heatflux2ENGOil_gain  InternalRulePriority=Speed  RndMeth=Simplest  InputSameDT=on
  Heat_flux_gain : Outport
  wires:
  T_ENGOil_degC/1 -> 1-D Lookup Table/1
  1-D Lookup Table/1 -> Heat_flux_gain/1

== system METI_CVT_Thermal_ver01_2015a/Vehicle/ENG_PNT/Coldstart_Heat_flux_gain_calc1 ==
  T_ENG_Cylinder_Head_degC : Inport
  1-D Lookup Table : Lookup_n-D  NumberOfTableDimensions=1  BreakpointsForDimension1=ENG_PNT_Heatflux2Cylinder_Head_gain_x_T_Coolant  Table=ENG_PNT_Heatflux2Cylinder_Head_gain  InternalRulePriority=Speed  RndMeth=Simplest  InputSameDT=on
  Heat_flux_gain : Outport
  wires:
  T_ENG_Cylinder_Head_degC/1 -> 1-D Lookup Table/1
  1-D Lookup Table/1 -> Heat_flux_gain/1

== system METI_CVT_Thermal_ver01_2015a/Vehicle/ENG_PNT/K->degC1 ==
  K : Inport
  Constant2 : Constant  Value=K2degC
  Sum : Sum  Inputs=++|
  degC : Outport
  wires:
  K/1 -> Sum/2
  Constant2/1 -> Sum/1
  Sum/1 -> degC/1

== system METI_CVT_Thermal_ver01_2015a/Vehicle/ENG_PNT/K->degC6 ==
  K : Inport
  Constant2 : Constant  Value=K2degC
  Sum : Sum  Inputs=++|
  degC : Outport
  wires:
  K/1 -> Sum/2
  Constant2/1 -> Sum/1
  Sum/1 -> degC/1

== system METI_CVT_Thermal_ver01_2015a/Vehicle/PTTH_PNT/DFTH_PNT ==
  note: T/Mブロックから
      | 受け取る熱量
  note: DFオイルの
      | 熱容量
  note: DFブロックの
      | 熱容量
  note: DFの損失が
      | DFオイルへの熱量
  note: エネルギーの
      | 向きの定義（仮）
      | →→→
  note: エネルギーの
      | 向きの定義（仮）
      | →→→
  note: エネルギーの
      | 向きの定義（仮）
      | →→→
  note: エネルギーの
      | 向きの定義（仮）
      | →→→
  note: エネルギーの
      | 向きの定義（仮）
      | →→→
  T_DF_Block_K : Inport
  PHI_DF_PNT_W : Inport  Port=2
  T_ATM_PNT_DF_K : Inport  Port=3
  DFBlock_Heat_Capacity : Subsystem
  DFOil2DFBlock_Heat_Resistance : Subsystem
  DFOil_Heat_Capacity : Subsystem
  ENGBlock2Air_Heat_Resistance : Subsystem
  TMBlock2DFBlock_Heat_Resistance : Subsystem
  Terminator : Terminator
  PHI_DF_Block_W : Outport
  PHI_DFTH_PNT_W : Outport  Port=2
  T_DFBlock_K : Outport  Port=3
  wires:
  DFOil_Heat_Capacity/1(T_DFOil2_K) -> DFOil2DFBlock_Heat_Resistance/1(T_DFOil_Resi2_K)
  DFOil2DFBlock_Heat_Resistance/1(PHI_DFOil_Resi2_W) -> DFOil_Heat_Capacity/1(PHI_DFOil2_W)
  DFBlock_Heat_Capacity/3(T_DFBlock1_K) -> DFOil2DFBlock_Heat_Resistance/2(T_DFBlock_Resi_K)
  DFOil2DFBlock_Heat_Resistance/2(PHI_DFBlock_Resi_W) -> DFBlock_Heat_Capacity/3(PHI_DFBlock1_W)
  ENGBlock2Air_Heat_Resistance/1(PHI_DFBlock_Resi_W) -> DFBlock_Heat_Capacity/1(PHI_DFBlock3_W)
  DFBlock_Heat_Capacity/2(T_DFBlock3_K) -> ENGBlock2Air_Heat_Resistance/1(T_DFBlock_Resi_K)
  T_ATM_PNT_DF_K/1 -> ENGBlock2Air_Heat_Resistance/2(T_DF_Air_Resi_K)
  ENGBlock2Air_Heat_Resistance/2(PHI_DF_Air_Resi_W) -> PHI_DFTH_PNT_W/1
  T_DF_Block_K/1 -> TMBlock2DFBlock_Heat_Resistance/2(T_TMBlock_Resi_K)
  TMBlock2DFBlock_Heat_Resistance/2(PHI_TMBlock_Resi_W) -> PHI_DF_Block_W/1
  TMBlock2DFBlock_Heat_Resistance/1(PHI_DFBlock_Resi_W) -> DFBlock_Heat_Capacity/2(PHI_DFBlock2_W)
  DFBlock_Heat_Capacity/1(T_DFBlock2_K) -> T_DFBlock_K/1, TMBlock2DFBlock_Heat_Resistance/1(T_DFBlock_Resi_K)
  DFOil_Heat_Capacity/2(T_DFOil1_K) -> Terminator/1
  PHI_DF_PNT_W/1 -> DFOil_Heat_Capacity/2(PHI_DFOil1_W)

== system METI_CVT_Thermal_ver01_2015a/Vehicle/PTTH_PNT/ENGTH_PNT ==
  note: エンジンオイル
      | 熱容量
  note: エンジン冷却水
      | 熱容量
  note: エンジンブロック
      | 熱容量
  note: 冷却水からラジエターへ
      | 放熱する熱量
  note: エネルギーの
      | 向きの定義（仮）
      | →→→
  note: エンジン燃焼室からシリンダヘッドへ
      | 放熱する熱量
  note: エンジンからエンジンオイルへ
      | 放熱する熱量
  note: エネルギーの
      | 向きの定義（仮）
      | →→→
  note: エネルギーの
      | 向きの定義（仮）
      | →→→
  note: エネルギーの
      | 向きの定義（仮）
      | →→→
  note: エネルギーの
      | 向きの定義（仮）
      | →→→
  note: エネルギーの
      | 向きの定義（仮）
      | →→→
  note: エネルギーの
      | 向きの定義（仮）
      | →→→
  note: エンジンブロックからT/Mブロックへ
      | 放熱する熱量
  note: シリンダヘッド
      | 熱容量
  note: エネルギーの
      | 向きの定義（仮）
      | →→→
  PHI_ENGBlock_W : Inport
  V_ENG_CNT_WP_V : Inport  Port=2
  PHI_ENG_PNT_Head_W : Inport  Port=3
  PHI_ENG_PNT_Oil_W : Inport  Port=4
  T_ATM_PNT_ENG_K : Inport  Port=5
  PHI_ENGCoolant_W : Inport  Port=6
  Coolant_Heat_Capacity : Subsystem
  Cylinder_Head2Coolant_Heat_Resistance : Subsystem
  ENGBlock2Air_Heat_Resistance : Subsystem
  ENGBlock2Coolant_Heat_Resistance : Subsystem
  ENGBlock_Heat_Capacity : Subsystem
  ENGOil2Coolant_Heat_Resistance : Subsystem
  ENGOil_Heat_Capacity : Subsystem
  ENGOil_Heat_Capacity1 : Subsystem
  Water_Pump : Subsystem
  T_ENGTH_PNT_Coolant_K : Outport
  T_ENG_Block_K : Outport  Port=2
  T_ENGTH_PNT_Oil_K : Outport  Port=3
  T_ENGTH_PNT_Head_K : Outport  Port=4
  PHI_ENGTH_PNT_W : Outport  Port=5
  wires:
  Coolant_Heat_Capacity/4(T_Coolant3_K) -> ENGOil2Coolant_Heat_Resistance/2(T_Coolant_Resi3_K)
  ENGOil2Coolant_Heat_Resistance/2(PHI_Coolant_Resi3_W) -> Coolant_Heat_Capacity/3(PHI_Coolant3_W)
  ENGOil_Heat_Capacity/1(T_ENGOil2_K) -> ENGOil2Coolant_Heat_Resistance/1(T_ENGOil_Resi2_K)
  ENGOil2Coolant_Heat_Resistance/1(PHI_ENGOil_Resi2_W) -> ENGOil_Heat_Capacity/1(PHI_ENGOil2_W)
  Coolant_Heat_Capacity/2(T_Coolant4_K) -> ENGBlock2Coolant_Heat_Resistance/1(T_Coolant_Resi4_K)
  ENGBlock2Coolant_Heat_Resistance/1(PHI_Coolant_Resi4_W) -> Coolant_Heat_Capacity/1(PHI_Coolant4_W)
  ENGBlock_Heat_Capacity/3(T_ENGBlock1_K) -> ENGBlock2Coolant_Heat_Resistance/2(T_ENGBlock_Resi1_K)
  ENGBlock2Coolant_Heat_Resistance/2(PHI_ENGBlock_Resi1_W) -> ENGBlock_Heat_Capacity/2(PHI_ENGBlock1_W)
  ENGBlock2Air_Heat_Resistance/1(PHI_ENGBlock_Resi3_W) -> ENGBlock_Heat_Capacity/1(PHI_ENGBlock3_W)
  ENGBlock_Heat_Capacity/1(T_ENGBlock3_K) -> ENGBlock2Air_Heat_Resistance/1(T_ENGBlock_Resi3_K)
  T_ATM_PNT_ENG_K/1 -> ENGBlock2Air_Heat_Resistance/2(T_ENG_Air_Resi1_K)
  ENGBlock2Air_Heat_Resistance/2(PHI_ENG_Air_Resi1_W) -> PHI_ENGTH_PNT_W/1
  Coolant_Heat_Capacity/3(T_Coolant2_K) -> T_ENGTH_PNT_Coolant_K/1  "T_ENGTH_PNT_Coolant_K"
  PHI_ENGCoolant_W/1 -> Coolant_Heat_Capacity/4(PHI_Coolant2_W)
  ENGBlock_Heat_Capacity/2(T_ENGBlock2_K) -> T_ENG_Block_K/1  "T_ENG_Block_K"
  PHI_ENGBlock_W/1 -> ENGBlock_Heat_Capacity/3(PHI_ENGBlock2_W)
  Cylinder_Head2Coolant_Heat_Resistance/1(PHI_Coolant_Resi1_W) -> Coolant_Heat_Capacity/2(PHI_Coolant1_W)
  Coolant_Heat_Capacity/1(T_Coolant1_K) -> Cylinder_Head2Coolant_Heat_Resistance/1(T_Coolant_Resi1_K)
  PHI_ENG_PNT_Oil_W/1 -> ENGOil_Heat_Capacity/2(PHI_ENGOil1_W)
  ENGOil_Heat_Capacity/2(T_ENGOil1_K) -> T_ENGTH_PNT_Oil_K/1  "T_ENGOil0_K"
  ENGOil_Heat_Capacity1/2(T_Cylinder_Head2_K) -> Cylinder_Head2Coolant_Heat_Resistance/3(T_Cylinder_Head_Resi2_K)
  Cylinder_Head2Coolant_Heat_Resistance/2(PHI_Cylinder_Head_Resi2_W) -> ENGOil_Heat_Capacity1/2(PHI_Cylinder_Head2_W)
  PHI_ENG_PNT_Head_W/1 -> ENGOil_Heat_Capacity1/1(PHI_Cylinder_Head1_W)
  ENGOil_Heat_Capacity1/1(T_Cylinder_Head1_K) -> T_ENGTH_PNT_Head_K/1  "T_Cylinder_Head0_K"
  Water_Pump/1(Qv_Coolant_m3ps) -> Cylinder_Head2Coolant_Heat_Resistance/2(Qv_Coolant_m3ps)
  V_ENG_CNT_WP_V/1 -> Water_Pump/1(ENG_PNT_Voltage_WP_V)

== system METI_CVT_Thermal_ver01_2015a/Vehicle/PTTH_PNT/K->degC ==
  K : Inport
  Constant2 : Constant  Value=K2degC
  Sum : Sum  Inputs=++|
  degC : Outport
  wires:
  K/1 -> Sum/2
  Constant2/1 -> Sum/1
  Sum/1 -> degC/1

== system METI_CVT_Thermal_ver01_2015a/Vehicle/PTTH_PNT/K->degC1 ==
  K : Inport
  Constant2 : Constant  Value=K2degC
  Sum : Sum  Inputs=++|
  degC : Outport
  wires:
  Sum/1 -> degC/1
  Constant2/1 -> Sum/1
  K/1 -> Sum/2

== system METI_CVT_Thermal_ver01_2015a/Vehicle/PTTH_PNT/K->degC2 ==
  K : Inport
  Constant2 : Constant  Value=K2degC
  Sum : Sum  Inputs=++|
  degC : Outport
  wires:
  K/1 -> Sum/2
  Constant2/1 -> Sum/1
  Sum/1 -> degC/1

== system METI_CVT_Thermal_ver01_2015a/Vehicle/PTTH_PNT/K->degC3 ==
  K : Inport
  Constant2 : Constant  Value=K2degC
  Sum : Sum  Inputs=++|
  degC : Outport
  wires:
  Sum/1 -> degC/1
  Constant2/1 -> Sum/1
  K/1 -> Sum/2

== system METI_CVT_Thermal_ver01_2015a/Vehicle/PTTH_PNT/K->degC4 ==
  K : Inport
  Constant2 : Constant  Value=K2degC
  Sum : Sum  Inputs=++|
  degC : Outport
  wires:
  K/1 -> Sum/2
  Constant2/1 -> Sum/1
  Sum/1 -> degC/1

== system METI_CVT_Thermal_ver01_2015a/Vehicle/PTTH_PNT/K->degC7 ==
  K : Inport
  Constant2 : Constant  Value=K2degC
  Sum : Sum  Inputs=++|
  degC : Outport
  wires:
  Sum/1 -> degC/1
  Constant2/1 -> Sum/1
  K/1 -> Sum/2

== system METI_CVT_Thermal_ver01_2015a/Vehicle/PTTH_PNT/RDTH_PNT ==
  note: サーモスタット
  note: エネルギーの
      | 向きの定義（仮）
      | →→→
  note: エネルギーの
      | 向きの定義（仮）
      | →→→
  v_VL_PNT_kmph : Inport
  RD_PNT_Voltage_RDFan_V : Inport  Port=2
  T_ENGTH_PNT_Coolant_K : Inport  Port=3
  T_ATM_PNT_RD_K : Inport  Port=4
  ENGBlock2Coolant_Heat_Resistance : Subsystem
  RDCoolant2Air_Heat_Resistance : Subsystem
  RDCoolant_Heat_Capacity : Subsystem
  RD_Core_Heat_Resi_Calc : Subsystem
  T_RDCoolant_degC : Outport
  PHI_RDTH_PNT_W : Outport  Port=2
  PHI_RD_Air_Resi_W : Outport  Port=3
  tag scope: RD_PNT_RDCore_Heat_Resi_KpW=global
  wires:
  RDCoolant_Heat_Capacity/1(T_RDCoolant1_K) -> ENGBlock2Coolant_Heat_Resistance/1(T_RDCoolant_Resi1_K)
  ENGBlock2Coolant_Heat_Resistance/1(PHI_RDCoolant_Resi1_W) -> RDCoolant_Heat_Capacity/1(PHI_RDCoolant1_W)
  T_ATM_PNT_RD_K/1 -> RDCoolant2Air_Heat_Resistance/1(T_RD_Air_Resi_K)
  RDCoolant2Air_Heat_Resistance/1(PHI_RD_Air_Resi1_W) -> PHI_RD_Air_Resi_W/1
  RDCoolant_Heat_Capacity/2(T_RDCoolant2_K) -> T_RDCoolant_degC/1, RDCoolant2Air_Heat_Resistance/3(T_RDCoolant_Resi2_K)
  RDCoolant2Air_Heat_Resistance/2(PHI_RDCoolant_Resi2_W) -> RDCoolant_Heat_Capacity/2(PHI_RDCoolant2_W)
  T_ENGTH_PNT_Coolant_K/1 -> ENGBlock2Coolant_Heat_Resistance/2(T_Thermostat_Resi1_K)
  ENGBlock2Coolant_Heat_Resistance/2(PHI_Thermostat_Resi1_W) -> PHI_RDTH_PNT_W/1
  RD_PNT_Voltage_RDFan_V/1 -> RD_Core_Heat_Resi_Calc/1(RD_PNT_Voltage_RDFan_V)
  v_VL_PNT_kmph/1 -> RD_Core_Heat_Resi_Calc/2(v_VL_PNT_kmph)
  RD_Core_Heat_Resi_Calc/1("RD_PNT_RDCore_Heat_Resi_KpW ") -> [RD_PNT_RDCore_Heat_Resi_KpW], RDCoolant2Air_Heat_Resistance/2("RD_PNT_RDCore_Heat_Resi_KpW ")

== system METI_CVT_Thermal_ver01_2015a/Vehicle/PTTH_PNT/TMTH_PNT ==
  note: CVTFの
      | 熱容量
  note: T/Mブロックの
      | 熱容量
  note: DFブロックへ
      | 放熱する熱量
  note: エンジンブロックから
      | 受け取る熱量
  note: CVTFからエンジン冷却水へ
      | 放熱する熱量
  note: T/Mの入力-出力が
      | CVTFへの熱量
  note: エネルギーの
      | 向きの定義（仮）
      | ←←←
  note: エネルギーの
      | 向きの定義（仮）
      | →→→
  note: エネルギーの
      | 向きの定義（仮）
      | →→→
  note: エネルギーの
      | 向きの定義（仮）
      | →→→
  note: エネルギーの
      | 向きの定義（仮）
      | →→→
  note: エネルギーの
      | 向きの定義（仮）
      | →→→
  note: エネルギーの
      | 向きの定義（仮）
      | →→→
  note: TMブロックからから大気へ
      | 放熱する熱量
  W_TM_Block0_W : Inport
  R_CVTF_warmer_tgt_KpW : Inport  Port=2
  PHI_TM_PNT_W : Inport  Port=3
  T_TM_Block_Resi_K : Inport  Port=4
  T_ENGTH_PNT_Coolant_K : Inport  Port=5
  T_ATM_PNT_TM_K : Inport  Port=6
  CVTF2Coolant_Heat_Resistance : Subsystem
  CVTF2TMBlock_Heat_Resistance : Subsystem
  CVTF_Heat_Capacity : Subsystem
  ENGBlock2TMBlock_Heat_Resistance : Subsystem
  TMBlock2Air_Heat_Resistance : Subsystem
  TMBlock_Heat_Capacity : Subsystem
  T_TMTH_PNT_CVTF1_K : Outport
  T_TM_Block0_K : Outport  Port=2
  PHI_TM_CVTF_Resi_W : Outport  Port=3
  T_TMTH_PNT_CVTF_K : Outport  Port=4
  PHI_ENGBlock_Resi2_W : Outport  Port=5
  PHI_TMTH_PNT_W : Outport  Port=6
  tag scope: R_CVTF_warmer_tgt_KpW=global
  wires:
  CVTF_Heat_Capacity/1(T_CVTF4_K) -> CVTF2TMBlock_Heat_Resistance/1(T_CVTF_Resi4_K)
  CVTF2TMBlock_Heat_Resistance/1(PHI_CVTF_Resi4_W) -> CVTF_Heat_Capacity/1(PHI_CVTF4_W)
  TMBlock_Heat_Capacity/4(T_TMBlock1_K) -> CVTF2TMBlock_Heat_Resistance/2(T_TMBlock_Resi1_K)
  CVTF2TMBlock_Heat_Resistance/2(PHI_TMBlock_Resi1_W) -> TMBlock_Heat_Capacity/3(PHI_TMBlock1_W)
  CVTF_Heat_Capacity/3(T_CVTF1_K) -> T_TMTH_PNT_CVTF_K/1, T_TMTH_PNT_CVTF1_K/1  "T_TMTH_PNT_CVTF_K"
  PHI_TM_PNT_W/1 -> CVTF_Heat_Capacity/2(PHI_CVTF1_W)
  TMBlock2Air_Heat_Resistance/1(PHI_TMBlock_Resi3_W) -> TMBlock_Heat_Capacity/1(PHI_TMBlock3_W)
  TMBlock_Heat_Capacity/2(T_TMBlock3_K) -> TMBlock2Air_Heat_Resistance/1(T_TMBlock_Resi3_K)
  T_ATM_PNT_TM_K/1 -> TMBlock2Air_Heat_Resistance/2(T_TM_Air_Resi1_K)
  TMBlock2Air_Heat_Resistance/2(PHI_TM_Air_Resi1_W) -> PHI_TMTH_PNT_W/1
  T_TM_Block_Resi_K/1 -> ENGBlock2TMBlock_Heat_Resistance/2(T_ENGBlock_Resi2_K)
  ENGBlock2TMBlock_Heat_Resistance/2(PHI_ENGBlock_Resi2_W) -> PHI_ENGBlock_Resi2_W/1  "PHI_ENGBlock_Resi2_W"
  CVTF_Heat_Capacity/2(T_CVTF2_K) -> CVTF2Coolant_Heat_Resistance/1(T_CVTF_Resi2_K)
  CVTF2Coolant_Heat_Resistance/2(PHI_CVTF_Resi2_W) -> CVTF_Heat_Capacity/3(PHI_CVT2_W)
  CVTF2Coolant_Heat_Resistance/1(PHI_Coolant_Resi2_W) -> PHI_TM_CVTF_Resi_W/1  "PHI_TM_CVTF_Resi_W"
  T_ENGTH_PNT_Coolant_K/1 -> CVTF2Coolant_Heat_Resistance/3(T_Coolant_Resi2_K)
  ENGBlock2TMBlock_Heat_Resistance/1(PHI_TMBlock_Resi2_W) -> TMBlock_Heat_Capacity/2(PHI_TMBlock2_W)
  TMBlock_Heat_Capacity/1(T_TMBlock2_K) -> ENGBlock2TMBlock_Heat_Resistance/1(T_TMBlock_Resi2_K)
  TMBlock_Heat_Capacity/3(T_TMBlock4_K) -> T_TM_Block0_K/1  "T_TM_Block0_degC"
  W_TM_Block0_W/1 -> TMBlock_Heat_Capacity/4(PHI_TMBlock4_W)
  R_CVTF_warmer_tgt_KpW/1 -> CVTF2Coolant_Heat_Resistance/2(R_CVTF_warmer_tgt_KpW), [R_CVTF_warmer_tgt_KpW]

== system METI_CVT_Thermal_ver01_2015a/Vehicle/TM_CNT/CVT_ECU ==
  per_throttle : Inport
  omg_pera : Inport  Port=2
  1-D Lookup Table : Lookup_n-D  NumberOfTableDimensions=1  BreakpointsForDimension1=TM_CNT_CVTpritgt_rpm_table_x_TVO  Table=TM_CNT_CVTpritgt_rpm_table  RndMeth=Simplest  InputSameDT=on
  Constant2 : Constant  Value=TM_CNT_CVT_radpmin_min_rpm
  Divide : Product  Inputs=*/
  Gain2 : Gain  Gain=TM_CNT_Gain_CVT_ECU
  HighestRatio : Constant  Value=TM_CNT_CVT_ratio_LL
  LowestRatio : Constant  Value=TM_CNT_CVT_ratio_UL
  MinMax : MinMax  Function=max  Inputs=2
  Saturation : Saturate  UpperLimit=TM_CNT_delta_CVT_ratio_UL  LowerLimit=TM_CNT_delta_CVT_ratio_LL
  Saturation Dynamic : simulink/Discontinuities/Saturation Dynamic  OutMin=[]  OutMax=[]  OutDataTypeStr=Inherit: Same as second input  OutDataType=fixdt(1, 16)  OutScaling=2^-10  DoSatur=off
  Sum : Sum  Inputs=|+-
  Sum1 : Sum  Inputs=|++
  Unit Delay : UnitDelay  InitialCondition=1  SampleTime=-1
  ratio_CVT : Outport
  wires:
  1-D Lookup Table/1 -> Divide/1
  Divide/1 -> Saturation Dynamic/2
  LowestRatio/1 -> Saturation Dynamic/1
  HighestRatio/1 -> Saturation Dynamic/3
  MinMax/1 -> Divide/2
  Saturation Dynamic/1 -> Sum/1
  Unit Delay/1 -> Sum1/2, Sum/2
  Sum1/1 -> ratio_CVT/1, Unit Delay/1
  Sum/1 -> Gain2/1
  Gain2/1 -> Saturation/1
  per_throttle/1 -> 1-D Lookup Table/1
  omg_pera/1 -> MinMax/2
  Saturation/1 -> Sum1/1
  Constant2/1 -> MinMax/1

== system METI_CVT_Thermal_ver01_2015a/Vehicle/TM_CNT/K->degC ==
  K : Inport
  Constant2 : Constant  Value=K2degC
  Sum : Sum  Inputs=++|
  degC : Outport
  wires:
  Sum/1 -> degC/1
  Constant2/1 -> Sum/1
  K/1 -> Sum/2

== system METI_CVT_Thermal_ver01_2015a/Vehicle/TM_CNT/K->degC1 ==
  K : Inport
  Constant2 : Constant  Value=K2degC
  Sum : Sum  Inputs=++|
  degC : Outport
  wires:
  K/1 -> Sum/2
  Constant2/1 -> Sum/1
  Sum/1 -> degC/1

== system METI_CVT_Thermal_ver01_2015a/Vehicle/TM_CNT/LockupClutch_ECU ==
  v_vehicle : Inport
  per_throttle : Inport  Port=2
  2-D Lookup Table : Lookup_n-D  BreakpointsForDimension1=TM_CNT_LU_slip_rpm_map_y_TVO  BreakpointsForDimension2=TM_CNT_LU_slip_rpm_map_x_speed_kmph  Table=TM_CNT_LU_slip_rpm_map  RndMeth=Simplest  InputSameDT=on
  Relay : Relay  OnSwitchValue=TM_CNT_LU_Clutch_RelayON_rpm  OffSwitchValue=TM_CNT_LU_Clutch_RelayOFF_rpm  OnOutputValue=0  OffOutputValue=1
  flag_Lockup : Outport
  omg_Slip_rpm : Outport  Port=2
  wires:
  v_vehicle/1 -> 2-D Lookup Table/2
  2-D Lookup Table/1 -> omg_Slip_rpm/1, Relay/1
  per_throttle/1 -> 2-D Lookup Table/1
  Relay/1 -> flag_Lockup/1

== system METI_CVT_Thermal_ver01_2015a/Vehicle/TM_CNT/WarmerECU ==
  note: ENG冷却水温＞CVTF温度
      | の時にこのマップを使用する
  note: CVTF温度が熱い時に
      | このマップを使用する
  T_TMTH_PNT_CVTF_dC : Inport
  T_ENG_Coolant_dC : Inport  Port=2
  1-D Lookup Table1 : Lookup_n-D  NumberOfTableDimensions=1  BreakpointsForDimension1=TM_CNT_CVTFwarmer_KpW_x_T_ENGCoolant  BeginIndexSearchUsingPreviousIndexResult=on  Table=TM_CNT_CVTFwarmer_KpW  ExtrapMethod=Clip  InternalRulePriority=Speed  RndMeth=Simplest  InputSameDT=on
  1-D Lookup Table2 : Lookup_n-D  NumberOfTableDimensions=1  BreakpointsForDimension1=TM_CNT_CVTFwarmer2_KpW_x_T_CVTF  BeginIndexSearchUsingPreviousIndexResult=on  Table=TM_CNT_CVTFwarmer2_KpW  ExtrapMethod=Clip  InternalRulePriority=Speed  RndMeth=Simplest  InputSameDT=on
  Add1 : Sum  Inputs=+-
  Compare To Zero1 : simulink/Logic and Bit Operations/Compare To Zero  relop=>  OutDataTypeStr=boolean
  Constant1 : Constant  Value=TM_CNT_CVTFwarmer_cold_Coolant_KpW
  MinMax : MinMax  Inputs=2
  Switch1 : Switch  Criteria=u2 > Threshold
  R_CVTF_warmer_tgt_KpW : Outport
  wires:
  MinMax/1 -> R_CVTF_warmer_tgt_KpW/1
  Add1/1 -> Compare To Zero1/1
  Compare To Zero1/1 -> Switch1/2
  1-D Lookup Table1/1 -> Switch1/1
  Constant1/1 -> Switch1/3
  T_ENG_Coolant_dC/1 -> 1-D Lookup Table1/1, Add1/1
  T_TMTH_PNT_CVTF_dC/1 -> 1-D Lookup Table2/1, Add1/2
  Switch1/1 -> MinMax/1
  1-D Lookup Table2/1 -> MinMax/2

== system METI_CVT_Thermal_ver01_2015a/Vehicle/TM_PNT/Flywheel ==
  trq_TM_PNT_in_Nm : Inport
  trq_TM_PNT_in_Nm1 : Inport  Port=2
  Divide : Product  Inputs=*/
  Inertia : Constant  Value=TM_PNT_Flywheel_Inertia_kgm2
  Integrator : Integrator  InitialCondition=TM_PNT_Flywheel_Init_radps  LimitOutput=on  LowerSaturationLimit=0
  P_cal : METI_Lib_vehicle_model/P_cal  Commented=on  Type_energy=回転運動  Type_output_energy=出力  Power_name=Po_  t_Workspace_Name=TM_PNT_Flywheel  P_VariableName=Po_TM_PNT_Flywheel  Across_VariableName=w_TM_PNT_Flywheel  Throgh_VariableName=tq_TM_PNT_Flywheel
  Sum : Sum  Inputs=|++
  Terminator : Terminator  Commented=on
  w_ENG_PNT_radps : Outport
  w_TM_PNT_in_radps : Outport  Port=2
  wires:
  Integrator/1 -> P_cal/1, w_TM_PNT_in_radps/1, w_ENG_PNT_radps/1
  trq_TM_PNT_in_Nm/1 -> Sum/1
  trq_TM_PNT_in_Nm1/1 -> Sum/2
  Inertia/1 -> Divide/2
  Sum/1 -> Divide/1, P_cal/2
  P_cal/1 -> Terminator/1
  Divide/1 -> Integrator/1

== system METI_CVT_Thermal_ver01_2015a/Vehicle/TM_PNT/Inertia ==
  trq_TM_PNT_out_Nm0 : Inport
  trq_TM_PNT_Nm : Inport  Port=2
  Divide : Product  Inputs=*/
  Inertia : Constant  Value=TM_PNT_Driveshaft_Inertia_kgm2
  Integrator : Integrator  InitialCondition=000*(2*pi)/60  LimitOutput=on  LowerSaturationLimit=0
  P_cal : METI_Lib_vehicle_model/P_cal  Type_energy=回転運動  Type_output_energy=出力  Power_name=Po_  t_Workspace_Name=TM_PNT_inertia_MECK  P_VariableName=Po_TM_PNT_inertia_MECK  Across_VariableName=w_TM_PNT_inertia_MECK  Throgh_VariableName=tq_TM_PNT_inertia_MECK
  Sum : Sum  Inputs=|++
  Terminator : Terminator
  w_TM_PNT_out_radps : Outport
  w_TM_PNT_out_radps0 : Outport  Port=2
  wires:
  Integrator/1 -> P_cal/1, w_TM_PNT_out_radps0/1, w_TM_PNT_out_radps/1
  Divide/1 -> Integrator/1
  trq_TM_PNT_out_Nm0/1 -> Sum/1
  trq_TM_PNT_Nm/1 -> Sum/2
  Inertia/1 -> Divide/2
  Sum/1 -> Divide/1, P_cal/2
  P_cal/1 -> Terminator/1

== system METI_CVT_Thermal_ver01_2015a/Vehicle/TM_PNT/K->degC6 ==
  K : Inport
  Constant2 : Constant  Value=K2degC
  Sum : Sum  Inputs=++|
  degC : Outport
  wires:
  K/1 -> Sum/2
  Constant2/1 -> Sum/1
  Sum/1 -> degC/1
